simulink model "pcss_example_1"  (Simulink 6.1)
settings: Solver=ode45  StartTime=0.0  StopTime=10000  RelTol=1e-3
libraries: simulink x1
settings Model: LastModifiedBy=pse
settings DataIOCC: MaxDataPoints=100000

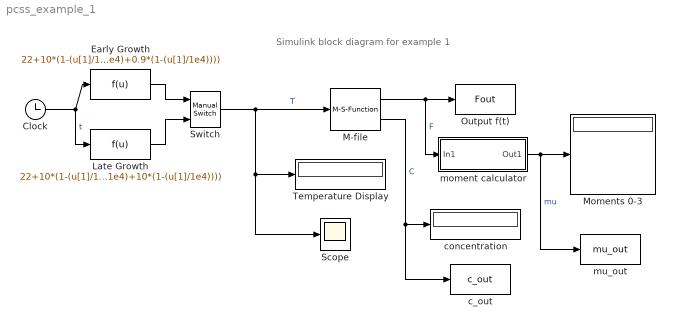
== system pcss_example_1 ==
  note: Simulink block diagram for example 1
  Clock : Clock
      settings: Decimation=10
  Early Growth : Fcn  Expr=22+10*(1-(u[1]/1e4)/((u[1]/1e4)+0.9*(1-(u[1]/1e4))))
  Late Growth : Fcn  Expr=22+10*(1-(u[1]/1e4)/((u[1]/1e4)+10*(1-(u[1]/1e4))))
  M-file : M-S-Function  MFile=PCSS  Parameters='pcss_ex_1'
  Moments 0-3 : Display
  Output f(t) : ToWorkspace  VariableName=Fout  SampleTime=-1  SaveFormat=Array
      settings: MaxDataPoints=1
  Scope : Scope
      settings: YMin=22  YMax=32
  Switch : simulink/Signal Routing/Manual Switch  sw=1  action=0
  Temperature Display : Display
  c_out : ToWorkspace  VariableName=c_out  SampleTime=-1  SaveFormat=Structure With Time
      settings: Decimation=10
  concentration : Display
  moment calculator : Subsystem  mask{dL='pcss_ex_1', mucalc=[0,1,2,3], mu_plot=[0 3], gf=100}
      mask prompts: dL "What is the value of dL?"; mucalc "Which moments should be calculated and output?"; mu_plot "Which moments should be graphed?"; gf "How often should the graph be updated?"
      mask Display:
      | port_label('input', 1, 'F')
      | port_label('output', 1, 'mu')
  mu_out : ToWorkspace  VariableName=mu_out  SampleTime=-1  SaveFormat=Structure With Time
      settings: Decimation=10
  wires:
  M-file/1 -> Output f(t)/1, moment calculator/1(In1)  "F"
  moment calculator/1(Out1) -> Moments 0-3/1, mu_out/1  "mu"
  Clock/1 -> Early Growth/1, Late Growth/1  "t"
  M-file/2 -> c_out/1, concentration/1  "C"
  Early Growth/1 -> Switch/1
  Late Growth/1 -> Switch/2
  Switch/1 -> M-file/1, Scope/1, Temperature Display/1  "T"

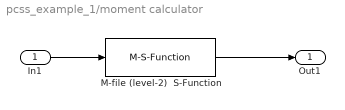
== system pcss_example_1/moment calculator ==
  In1 : Inport  Port=1  LatchInput=off
  M-file (level-2)  S-Function : M-S-Function  MFile=mu_calc  Parameters=dL,mucalc,mu_plot,gf
  Out1 : Outport
  wires:
  M-file (level-2)  S-Function/1 -> Out1/1
  In1/1 -> M-file (level-2)  S-Function/1
